simulink model "chap8_24sim"  (Simulink 7.7)
settings: Solver=ode45  StartTime=0  StopTime=2  FixedStep=0.001  RelTol=1e-3
libraries: simulink x1
settings Model: Creator=hp  LastModifiedBy=ljk
settings DataIOCC: SignalLoggingName=sigsOut
settings OptimizationCC: InitFltsAndDblsToZero=on
settings DebuggingCC: SaveWithParameterizedLinksMsg=none  SignalResolutionControl=TryResolveAllWithWarning  SolverPrmCheckMsg=none  MultiTaskDSMMsg=warning  MultiTaskCondExecSysMsg=none  StrictBusMsg=Warning
settings HardwareCC: TargetUnknown=on
settings RTWCC: IncludeERTFirstTime=on
settings GRTTargetCC: TargetFcnLib=ansi_tfl_tmw.mat

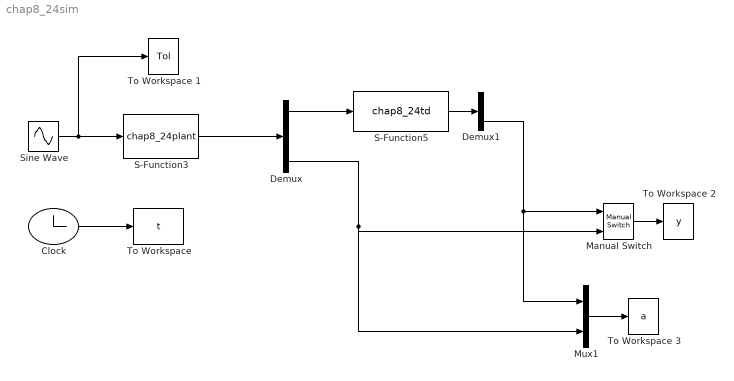
== system chap8_24sim ==
  Clock : Clock
      settings: Decimation=10
  Demux : Demux  Outputs=3
  Demux1 : Demux  Outputs=3
  Manual Switch : simulink/Signal Routing/Manual Switch  SystemSampleTime=-1  sw=0  action=0  varsize=off
  Mux1 : Mux  Inputs=2
  S-Function3 : S-Function  FunctionName=chap8_24plant  EnableBusSupport=off
  S-Function5 : S-Function  FunctionName=chap8_24td  EnableBusSupport=off
  Sine Wave : Sin  Frequency=2*pi  SampleTime=0
  To Workspace : ToWorkspace  VariableName=t  SampleTime=-1  SaveFormat=Array
  To Workspace 1 : ToWorkspace  VariableName=Tol  SampleTime=-1  SaveFormat=Array
  To Workspace 2 : ToWorkspace  VariableName=y  SampleTime=-1  SaveFormat=Array
  To Workspace 3 : ToWorkspace  VariableName=a  SampleTime=-1  SaveFormat=Array
  wires:
  Clock/1 -> To Workspace/1
  Sine Wave/1 -> S-Function3/1, To Workspace 1/1
  S-Function3/1 -> Demux/1
  Demux/1 -> S-Function5/1
  S-Function5/1 -> Demux1/1
  Mux1/1 -> To Workspace 3/1
  Manual Switch/1 -> To Workspace 2/1
  Demux/3 -> Manual Switch/2, Mux1/2
  Demux1/3 -> Manual Switch/1, Mux1/1
